simulink library "EmE_MBD_Blockset"  (R2018a)
settings: Solver=ode1  StartTime=0.0  StopTime=Inf  FixedStep=0.001  RelTol=1e-3  EnableMultiTasking=on
PostLoadFcn:
  | , if any(exist('dsrtsu_mdlpostloadfcn', 'file') == [2, 3, 6]), try dsrtsu_mdlpostloadfcn('Execute', bdroot); catch fprintf('Error in PostLoadFcn (dsrtsu_mdlpostloadfcn) for model "%s":\n %s\n', bdroot, lasterr); end, end,
undefined symbols (not defined in the file or in its folder): ENUM_TSC1_CONTROL_PURPOSE_T, gcbh, GLB_SWITCH_T
libraries: simulink x237, $bdroot x115, simulink_need_slupdate x26, MotoHawk_lib x13, simulink_extras x3
(part 7 of 11)

== system EmE_MBD_Blockset/User-Defined Functions/Snoop/CCP_ETC_SS1/Signal Data Pairing/Update Signal4 ==
  note: Configured signal information
  note: Memory address currently being configured
  PID : Inport
  Offset : Inport  Port=2
  ResetDAQ : Inport  Port=3
  Memory_Address : Inport  Port=4
  Signal_Info : Inport  Port=5
  Bus Creator : BusCreator  Inputs=6
  Bus Selector1 : BusSelector  OutputSignals=Signal_Address,Signal_Type,Signal_Conversion
  Detect Rise Positive : simulink/Logic and Bit Operations/Detect Rise Positive  vinit=0  InputProcessing=Inherited  OutDataTypeStr=uint8
  Latch w Update : Subsystem
  Latch w Update1 : Subsystem
  RS Flop-Flop Rp : Subsystem
      mask help: RS flip-flop with priority on R
  Relational Operator2 : RelationalOperator  Operator===  OutDataTypeStr=boolean  RndMeth=Nearest
  Reset Logic : Subsystem
  Terminator : Terminator
  Signal_Data_Updated : Outport
  wires:
  [PID] -> Reset Logic/1(CurrentPID)
  ResetDAQ/1 -> Reset Logic/2(ResetDAQ)
  Reset Logic/1(Reset) -> RS Flop-Flop Rp/1(Rp)
  Bus Selector1/1 -> Relational Operator2/2, Bus Creator/4  "<Signal_Address>"
  Bus Selector1/2 -> Bus Creator/5  "<Signal_Type>"
  Relational Operator2/1 -> Detect Rise Positive/1, RS Flop-Flop Rp/2(S)  "F_Signal_Defined"
  Memory_Address/1 -> Relational Operator2/1
  Signal_Info/1 -> Bus Selector1/1
  Bus Creator/1 -> Signal_Data_Updated/1
  Latch w Update/1(Latched) -> [PID], Bus Creator/1  "PID"
  Latch w Update1/1(Latched) -> Bus Creator/2  "Offset"
  Offset/1 -> Latch w Update1/2(In)
  PID/1 -> Latch w Update/2(In)
  Bus Selector1/3 -> Bus Creator/6  "<Signal_Conversion>"
  Detect Rise Positive/1 -> Latch w Update/1(f_update), Latch w Update1/1(f_update)
  RS Flop-Flop Rp/1(Q) -> Bus Creator/3  "F_Defined"
  RS Flop-Flop Rp/2(!Q) -> Terminator/1

== system EmE_MBD_Blockset/User-Defined Functions/Snoop/CCP_ETC_SS1/Signal Data Pairing/Update Signal5 ==
  note: Configured signal information
  note: Memory address currently being configured
  PID : Inport
  Offset : Inport  Port=2
  ResetDAQ : Inport  Port=3
  Memory_Address : Inport  Port=4
  Signal_Info : Inport  Port=5
  Bus Creator : BusCreator  Inputs=6
  Bus Selector1 : BusSelector  OutputSignals=Signal_Address,Signal_Type,Signal_Conversion
  Detect Rise Positive : simulink/Logic and Bit Operations/Detect Rise Positive  vinit=0  InputProcessing=Inherited  OutDataTypeStr=uint8
  Latch w Update : Subsystem
  Latch w Update1 : Subsystem
  RS Flop-Flop Rp : Subsystem
      mask help: RS flip-flop with priority on R
  Relational Operator2 : RelationalOperator  Operator===  OutDataTypeStr=boolean  RndMeth=Nearest
  Reset Logic : Subsystem
  Terminator : Terminator
  Signal_Data_Updated : Outport
  wires:
  [PID] -> Reset Logic/1(CurrentPID)
  ResetDAQ/1 -> Reset Logic/2(ResetDAQ)
  Reset Logic/1(Reset) -> RS Flop-Flop Rp/1(Rp)
  Bus Selector1/1 -> Relational Operator2/2, Bus Creator/4  "<Signal_Address>"
  Bus Selector1/2 -> Bus Creator/5  "<Signal_Type>"
  Relational Operator2/1 -> Detect Rise Positive/1, RS Flop-Flop Rp/2(S)  "F_Signal_Defined"
  Memory_Address/1 -> Relational Operator2/1
  Signal_Info/1 -> Bus Selector1/1
  Bus Creator/1 -> Signal_Data_Updated/1
  Latch w Update/1(Latched) -> [PID], Bus Creator/1  "PID"
  Latch w Update1/1(Latched) -> Bus Creator/2  "Offset"
  Offset/1 -> Latch w Update1/2(In)
  PID/1 -> Latch w Update/2(In)
  Bus Selector1/3 -> Bus Creator/6  "<Signal_Conversion>"
  Detect Rise Positive/1 -> Latch w Update/1(f_update), Latch w Update1/1(f_update)
  RS Flop-Flop Rp/1(Q) -> Bus Creator/3  "F_Defined"
  RS Flop-Flop Rp/2(!Q) -> Terminator/1

== system EmE_MBD_Blockset/User-Defined Functions/Snoop/CCP_ETC_SS1/Signal Data Pairing/Update Signal6 ==
  note: Configured signal information
  note: Memory address currently being configured
  PID : Inport
  Offset : Inport  Port=2
  ResetDAQ : Inport  Port=3
  Memory_Address : Inport  Port=4
  Signal_Info : Inport  Port=5
  Bus Creator : BusCreator  Inputs=6
  Bus Selector1 : BusSelector  OutputSignals=Signal_Address,Signal_Type,Signal_Conversion
  Detect Rise Positive : simulink/Logic and Bit Operations/Detect Rise Positive  vinit=0  InputProcessing=Inherited  OutDataTypeStr=uint8
  Latch w Update : Subsystem
  Latch w Update1 : Subsystem
  RS Flop-Flop Rp : Subsystem
      mask help: RS flip-flop with priority on R
  Relational Operator2 : RelationalOperator  Operator===  OutDataTypeStr=boolean  RndMeth=Nearest
  Reset Logic : Subsystem
  Terminator : Terminator
  Signal_Data_Updated : Outport
  wires:
  [PID] -> Reset Logic/1(CurrentPID)
  ResetDAQ/1 -> Reset Logic/2(ResetDAQ)
  Reset Logic/1(Reset) -> RS Flop-Flop Rp/1(Rp)
  Bus Selector1/1 -> Relational Operator2/2, Bus Creator/4  "<Signal_Address>"
  Bus Selector1/2 -> Bus Creator/5  "<Signal_Type>"
  Relational Operator2/1 -> Detect Rise Positive/1, RS Flop-Flop Rp/2(S)  "F_Signal_Defined"
  Memory_Address/1 -> Relational Operator2/1
  Signal_Info/1 -> Bus Selector1/1
  Bus Creator/1 -> Signal_Data_Updated/1
  Latch w Update/1(Latched) -> [PID], Bus Creator/1  "PID"
  Latch w Update1/1(Latched) -> Bus Creator/2  "Offset"
  Offset/1 -> Latch w Update1/2(In)
  PID/1 -> Latch w Update/2(In)
  Bus Selector1/3 -> Bus Creator/6  "<Signal_Conversion>"
  Detect Rise Positive/1 -> Latch w Update/1(f_update), Latch w Update1/1(f_update)
  RS Flop-Flop Rp/1(Q) -> Bus Creator/3  "F_Defined"
  RS Flop-Flop Rp/2(!Q) -> Terminator/1

== system EmE_MBD_Blockset/User-Defined Functions/Snoop/CCP_ETC_SS1/Signal Data Pairing/Update Signal7 ==
  note: Configured signal information
  note: Memory address currently being configured
  PID : Inport
  Offset : Inport  Port=2
  ResetDAQ : Inport  Port=3
  Memory_Address : Inport  Port=4
  Signal_Info : Inport  Port=5
  Bus Creator : BusCreator  Inputs=6
  Bus Selector1 : BusSelector  OutputSignals=Signal_Address,Signal_Type,Signal_Conversion
  Detect Rise Positive : simulink/Logic and Bit Operations/Detect Rise Positive  vinit=0  InputProcessing=Inherited  OutDataTypeStr=uint8
  Latch w Update : Subsystem
  Latch w Update1 : Subsystem
  RS Flop-Flop Rp : Subsystem
      mask help: RS flip-flop with priority on R
  Relational Operator2 : RelationalOperator  Operator===  OutDataTypeStr=boolean  RndMeth=Nearest
  Reset Logic : Subsystem
  Terminator : Terminator
  Signal_Data_Updated : Outport
  wires:
  [PID] -> Reset Logic/1(CurrentPID)
  ResetDAQ/1 -> Reset Logic/2(ResetDAQ)
  Reset Logic/1(Reset) -> RS Flop-Flop Rp/1(Rp)
  Bus Selector1/1 -> Relational Operator2/2, Bus Creator/4  "<Signal_Address>"
  Bus Selector1/2 -> Bus Creator/5  "<Signal_Type>"
  Relational Operator2/1 -> Detect Rise Positive/1, RS Flop-Flop Rp/2(S)  "F_Signal_Defined"
  Memory_Address/1 -> Relational Operator2/1
  Signal_Info/1 -> Bus Selector1/1
  Bus Creator/1 -> Signal_Data_Updated/1
  Latch w Update/1(Latched) -> [PID], Bus Creator/1  "PID"
  Latch w Update1/1(Latched) -> Bus Creator/2  "Offset"
  Offset/1 -> Latch w Update1/2(In)
  PID/1 -> Latch w Update/2(In)
  Bus Selector1/3 -> Bus Creator/6  "<Signal_Conversion>"
  Detect Rise Positive/1 -> Latch w Update/1(f_update), Latch w Update1/1(f_update)
  RS Flop-Flop Rp/1(Q) -> Bus Creator/3  "F_Defined"
  RS Flop-Flop Rp/2(!Q) -> Terminator/1

== system EmE_MBD_Blockset/User-Defined Functions/Snoop/CCP_ETC_SS1/Signal Data Pairing/Update Signal8 ==
  note: Configured signal information
  note: Memory address currently being configured
  PID : Inport
  Offset : Inport  Port=2
  ResetDAQ : Inport  Port=3
  Memory_Address : Inport  Port=4
  Signal_Info : Inport  Port=5
  Bus Creator : BusCreator  Inputs=6
  Bus Selector1 : BusSelector  OutputSignals=Signal_Address,Signal_Type,Signal_Conversion
  Detect Rise Positive : simulink/Logic and Bit Operations/Detect Rise Positive  vinit=0  InputProcessing=Inherited  OutDataTypeStr=uint8
  Latch w Update : Subsystem
  Latch w Update1 : Subsystem
  RS Flop-Flop Rp : Subsystem
      mask help: RS flip-flop with priority on R
  Relational Operator2 : RelationalOperator  Operator===  OutDataTypeStr=boolean  RndMeth=Nearest
  Reset Logic : Subsystem
  Terminator : Terminator
  Signal_Data_Updated : Outport
  wires:
  [PID] -> Reset Logic/1(CurrentPID)
  ResetDAQ/1 -> Reset Logic/2(ResetDAQ)
  Reset Logic/1(Reset) -> RS Flop-Flop Rp/1(Rp)
  Bus Selector1/1 -> Relational Operator2/2, Bus Creator/4  "<Signal_Address>"
  Bus Selector1/2 -> Bus Creator/5  "<Signal_Type>"
  Relational Operator2/1 -> Detect Rise Positive/1, RS Flop-Flop Rp/2(S)  "F_Signal_Defined"
  Memory_Address/1 -> Relational Operator2/1
  Signal_Info/1 -> Bus Selector1/1
  Bus Creator/1 -> Signal_Data_Updated/1
  Latch w Update/1(Latched) -> [PID], Bus Creator/1  "PID"
  Latch w Update1/1(Latched) -> Bus Creator/2  "Offset"
  Offset/1 -> Latch w Update1/2(In)
  PID/1 -> Latch w Update/2(In)
  Bus Selector1/3 -> Bus Creator/6  "<Signal_Conversion>"
  Detect Rise Positive/1 -> Latch w Update/1(f_update), Latch w Update1/1(f_update)
  RS Flop-Flop Rp/1(Q) -> Bus Creator/3  "F_Defined"
  RS Flop-Flop Rp/2(!Q) -> Terminator/1

== system EmE_MBD_Blockset/User-Defined Functions/Snoop/CCP_ETC_SS1/Signal Data Pairing/Update Signal9 ==
  note: Configured signal information
  note: Memory address currently being configured
  PID : Inport
  Offset : Inport  Port=2
  ResetDAQ : Inport  Port=3
  Memory_Address : Inport  Port=4
  Signal_Info : Inport  Port=5
  Bus Creator : BusCreator  Inputs=6
  Bus Selector1 : BusSelector  OutputSignals=Signal_Address,Signal_Type,Signal_Conversion
  Detect Rise Positive : simulink/Logic and Bit Operations/Detect Rise Positive  vinit=0  InputProcessing=Inherited  OutDataTypeStr=uint8
  Latch w Update : Subsystem
  Latch w Update1 : Subsystem
  RS Flop-Flop Rp : Subsystem
      mask help: RS flip-flop with priority on R
  Relational Operator2 : RelationalOperator  Operator===  OutDataTypeStr=boolean  RndMeth=Nearest
  Reset Logic : Subsystem
  Terminator : Terminator
  Signal_Data_Updated : Outport
  wires:
  [PID] -> Reset Logic/1(CurrentPID)
  ResetDAQ/1 -> Reset Logic/2(ResetDAQ)
  Reset Logic/1(Reset) -> RS Flop-Flop Rp/1(Rp)
  Bus Selector1/1 -> Relational Operator2/2, Bus Creator/4  "<Signal_Address>"
  Bus Selector1/2 -> Bus Creator/5  "<Signal_Type>"
  Relational Operator2/1 -> Detect Rise Positive/1, RS Flop-Flop Rp/2(S)  "F_Signal_Defined"
  Memory_Address/1 -> Relational Operator2/1
  Signal_Info/1 -> Bus Selector1/1
  Bus Creator/1 -> Signal_Data_Updated/1
  Latch w Update/1(Latched) -> [PID], Bus Creator/1  "PID"
  Latch w Update1/1(Latched) -> Bus Creator/2  "Offset"
  Offset/1 -> Latch w Update1/2(In)
  PID/1 -> Latch w Update/2(In)
  Bus Selector1/3 -> Bus Creator/6  "<Signal_Conversion>"
  Detect Rise Positive/1 -> Latch w Update/1(f_update), Latch w Update1/1(f_update)
  RS Flop-Flop Rp/1(Q) -> Bus Creator/3  "F_Defined"
  RS Flop-Flop Rp/2(!Q) -> Terminator/1

== system EmE_MBD_Blockset/User-Defined Functions/Snoop/CCP_ETC_SS2/CCP_Parameter_Decode/Decode_Signal1 ==
  PID : Inport
  Data : Inport  Port=2
  Signal_Info : Inport  Port=3
  Bus Selector : BusSelector  OutputSignals=Offset,Signal_Address,Signal_Type,Signal_Conversion,PID,F_Defined
  Isolate Data : Subsystem
  Relational Operator : RelationalOperator  Operator===  OutDataTypeStr=boolean  RndMeth=Nearest
  Signal Decode : Subsystem
  Switch2 : Switch  Criteria=u2 ~= 0
  Terminator : Terminator
  Terminator1 : Terminator
  Unit Delay : UnitDelay  SampleTime=-1
  Signal : Outport
  wires:
  Bus Selector/2 -> Terminator/1  "<Signal_Address>"
  Switch2/1 -> Signal/1, Unit Delay/1
  Bus Selector/6 -> Terminator1/1  "<F_Defined>"
  Signal Decode/1(Out1) -> Switch2/1
  Unit Delay/1 -> Switch2/3
  Bus Selector/1 -> Isolate Data/1(Offset)  "<Offset>"
  PID/1 -> Relational Operator/2
  Relational Operator/1 -> Switch2/2
  Data/1 -> Isolate Data/2(Data)
  Bus Selector/5 -> Relational Operator/1  "<PID>"
  Bus Selector/3 -> Signal Decode/2(Type), Isolate Data/3(Type)  "<Signal_Type>"
  Bus Selector/4 -> Signal Decode/3(Coversion)  "<Signal_Conversion>"
  Signal_Info/1 -> Bus Selector/1
  Isolate Data/1(Raw32) -> Signal Decode/1(Raw32)

== system EmE_MBD_Blockset/User-Defined Functions/Snoop/CCP_ETC_SS2/CCP_Parameter_Decode/Decode_Signal10 ==
  PID : Inport
  Data : Inport  Port=2
  Signal_Info : Inport  Port=3
  Bus Selector : BusSelector  OutputSignals=Offset,Signal_Address,Signal_Type,Signal_Conversion,PID,F_Defined
  Isolate Data : Subsystem
  Relational Operator : RelationalOperator  Operator===  OutDataTypeStr=boolean  RndMeth=Nearest
  Signal Decode : Subsystem
  Switch2 : Switch  Criteria=u2 ~= 0
  Terminator : Terminator
  Terminator1 : Terminator
  Unit Delay : UnitDelay  SampleTime=-1
  Signal : Outport
  wires:
  Isolate Data/1(Raw32) -> Signal Decode/1(Raw32)
  Signal_Info/1 -> Bus Selector/1
  Bus Selector/4 -> Signal Decode/3(Coversion)  "<Signal_Conversion>"
  Bus Selector/3 -> Isolate Data/3(Type), Signal Decode/2(Type)  "<Signal_Type>"
  Bus Selector/5 -> Relational Operator/1  "<PID>"
  Data/1 -> Isolate Data/2(Data)
  Relational Operator/1 -> Switch2/2
  PID/1 -> Relational Operator/2
  Bus Selector/1 -> Isolate Data/1(Offset)  "<Offset>"
  Unit Delay/1 -> Switch2/3
  Signal Decode/1(Out1) -> Switch2/1
  Bus Selector/6 -> Terminator1/1  "<F_Defined>"
  Switch2/1 -> Unit Delay/1, Signal/1
  Bus Selector/2 -> Terminator/1  "<Signal_Address>"

== system EmE_MBD_Blockset/User-Defined Functions/Snoop/CCP_ETC_SS2/CCP_Parameter_Decode/Decode_Signal11 ==
  PID : Inport
  Data : Inport  Port=2
  Signal_Info : Inport  Port=3
  Bus Selector : BusSelector  OutputSignals=Offset,Signal_Address,Signal_Type,Signal_Conversion,PID,F_Defined
  Isolate Data : Subsystem
  Relational Operator : RelationalOperator  Operator===  OutDataTypeStr=boolean  RndMeth=Nearest
  Signal Decode : Subsystem
  Switch2 : Switch  Criteria=u2 ~= 0
  Terminator : Terminator
  Terminator1 : Terminator
  Unit Delay : UnitDelay  SampleTime=-1
  Signal : Outport
  wires:
  Bus Selector/2 -> Terminator/1  "<Signal_Address>"
  Switch2/1 -> Signal/1, Unit Delay/1
  Bus Selector/6 -> Terminator1/1  "<F_Defined>"
  Signal Decode/1(Out1) -> Switch2/1
  Unit Delay/1 -> Switch2/3
  Bus Selector/1 -> Isolate Data/1(Offset)  "<Offset>"
  PID/1 -> Relational Operator/2
  Relational Operator/1 -> Switch2/2
  Data/1 -> Isolate Data/2(Data)
  Bus Selector/5 -> Relational Operator/1  "<PID>"
  Bus Selector/3 -> Signal Decode/2(Type), Isolate Data/3(Type)  "<Signal_Type>"
  Bus Selector/4 -> Signal Decode/3(Coversion)  "<Signal_Conversion>"
  Signal_Info/1 -> Bus Selector/1
  Isolate Data/1(Raw32) -> Signal Decode/1(Raw32)

== system EmE_MBD_Blockset/User-Defined Functions/Snoop/CCP_ETC_SS2/CCP_Parameter_Decode/Decode_Signal12 ==
  PID : Inport
  Data : Inport  Port=2
  Signal_Info : Inport  Port=3
  Bus Selector : BusSelector  OutputSignals=Offset,Signal_Address,Signal_Type,Signal_Conversion,PID,F_Defined
  Isolate Data : Subsystem
  Relational Operator : RelationalOperator  Operator===  OutDataTypeStr=boolean  RndMeth=Nearest
  Signal Decode : Subsystem
  Switch2 : Switch  Criteria=u2 ~= 0
  Terminator : Terminator
  Terminator1 : Terminator
  Unit Delay : UnitDelay  SampleTime=-1
  Signal : Outport
  wires:
  Isolate Data/1(Raw32) -> Signal Decode/1(Raw32)
  Signal_Info/1 -> Bus Selector/1
  Bus Selector/4 -> Signal Decode/3(Coversion)  "<Signal_Conversion>"
  Bus Selector/3 -> Isolate Data/3(Type), Signal Decode/2(Type)  "<Signal_Type>"
  Bus Selector/5 -> Relational Operator/1  "<PID>"
  Data/1 -> Isolate Data/2(Data)
  Relational Operator/1 -> Switch2/2
  PID/1 -> Relational Operator/2
  Bus Selector/1 -> Isolate Data/1(Offset)  "<Offset>"
  Unit Delay/1 -> Switch2/3
  Signal Decode/1(Out1) -> Switch2/1
  Bus Selector/6 -> Terminator1/1  "<F_Defined>"
  Switch2/1 -> Unit Delay/1, Signal/1
  Bus Selector/2 -> Terminator/1  "<Signal_Address>"

== system EmE_MBD_Blockset/User-Defined Functions/Snoop/CCP_ETC_SS2/CCP_Parameter_Decode/Decode_Signal2 ==
  PID : Inport
  Data : Inport  Port=2
  Signal_Info : Inport  Port=3
  Bus Selector : BusSelector  OutputSignals=Offset,Signal_Address,Signal_Type,Signal_Conversion,PID,F_Defined
  Isolate Data : Subsystem
  Relational Operator : RelationalOperator  Operator===  OutDataTypeStr=boolean  RndMeth=Nearest
  Signal Decode : Subsystem
  Switch2 : Switch  Criteria=u2 ~= 0
  Terminator : Terminator
  Terminator1 : Terminator
  Unit Delay : UnitDelay  SampleTime=-1
  Signal : Outport
  wires:
  Isolate Data/1(Raw32) -> Signal Decode/1(Raw32)
  Signal_Info/1 -> Bus Selector/1
  Bus Selector/4 -> Signal Decode/3(Coversion)  "<Signal_Conversion>"
  Bus Selector/3 -> Isolate Data/3(Type), Signal Decode/2(Type)  "<Signal_Type>"
  Bus Selector/5 -> Relational Operator/1  "<PID>"
  Data/1 -> Isolate Data/2(Data)
  Relational Operator/1 -> Switch2/2
  PID/1 -> Relational Operator/2
  Bus Selector/1 -> Isolate Data/1(Offset)  "<Offset>"
  Unit Delay/1 -> Switch2/3
  Signal Decode/1(Out1) -> Switch2/1
  Bus Selector/6 -> Terminator1/1  "<F_Defined>"
  Switch2/1 -> Unit Delay/1, Signal/1
  Bus Selector/2 -> Terminator/1  "<Signal_Address>"

== system EmE_MBD_Blockset/User-Defined Functions/Snoop/CCP_ETC_SS2/CCP_Parameter_Decode/Decode_Signal3 ==
  PID : Inport
  Data : Inport  Port=2
  Signal_Info : Inport  Port=3
  Bus Selector : BusSelector  OutputSignals=Offset,Signal_Address,Signal_Type,Signal_Conversion,PID,F_Defined
  Isolate Data : Subsystem
  Relational Operator : RelationalOperator  Operator===  OutDataTypeStr=boolean  RndMeth=Nearest
  Signal Decode : Subsystem
  Switch2 : Switch  Criteria=u2 ~= 0
  Terminator : Terminator
  Terminator1 : Terminator
  Unit Delay : UnitDelay  SampleTime=-1
  Signal : Outport
  wires:
  Bus Selector/2 -> Terminator/1  "<Signal_Address>"
  Switch2/1 -> Signal/1, Unit Delay/1
  Bus Selector/6 -> Terminator1/1  "<F_Defined>"
  Signal Decode/1(Out1) -> Switch2/1
  Unit Delay/1 -> Switch2/3
  Bus Selector/1 -> Isolate Data/1(Offset)  "<Offset>"
  PID/1 -> Relational Operator/2
  Relational Operator/1 -> Switch2/2
  Data/1 -> Isolate Data/2(Data)
  Bus Selector/5 -> Relational Operator/1  "<PID>"
  Bus Selector/3 -> Signal Decode/2(Type), Isolate Data/3(Type)  "<Signal_Type>"
  Bus Selector/4 -> Signal Decode/3(Coversion)  "<Signal_Conversion>"
  Signal_Info/1 -> Bus Selector/1
  Isolate Data/1(Raw32) -> Signal Decode/1(Raw32)

== system EmE_MBD_Blockset/User-Defined Functions/Snoop/CCP_ETC_SS2/CCP_Parameter_Decode/Decode_Signal4 ==
  PID : Inport
  Data : Inport  Port=2
  Signal_Info : Inport  Port=3
  Bus Selector : BusSelector  OutputSignals=Offset,Signal_Address,Signal_Type,Signal_Conversion,PID,F_Defined
  Isolate Data : Subsystem
  Relational Operator : RelationalOperator  Operator===  OutDataTypeStr=boolean  RndMeth=Nearest
  Signal Decode : Subsystem
  Switch2 : Switch  Criteria=u2 ~= 0
  Terminator : Terminator
  Terminator1 : Terminator
  Unit Delay : UnitDelay  SampleTime=-1
  Signal : Outport
  wires:
  Isolate Data/1(Raw32) -> Signal Decode/1(Raw32)
  Signal_Info/1 -> Bus Selector/1
  Bus Selector/4 -> Signal Decode/3(Coversion)  "<Signal_Conversion>"
  Bus Selector/3 -> Isolate Data/3(Type), Signal Decode/2(Type)  "<Signal_Type>"
  Bus Selector/5 -> Relational Operator/1  "<PID>"
  Data/1 -> Isolate Data/2(Data)
  Relational Operator/1 -> Switch2/2
  PID/1 -> Relational Operator/2
  Bus Selector/1 -> Isolate Data/1(Offset)  "<Offset>"
  Unit Delay/1 -> Switch2/3
  Signal Decode/1(Out1) -> Switch2/1
  Bus Selector/6 -> Terminator1/1  "<F_Defined>"
  Switch2/1 -> Unit Delay/1, Signal/1
  Bus Selector/2 -> Terminator/1  "<Signal_Address>"

== system EmE_MBD_Blockset/User-Defined Functions/Snoop/CCP_ETC_SS2/CCP_Parameter_Decode/Decode_Signal5 ==
  PID : Inport
  Data : Inport  Port=2
  Signal_Info : Inport  Port=3
  Bus Selector : BusSelector  OutputSignals=Offset,Signal_Address,Signal_Type,Signal_Conversion,PID,F_Defined
  Isolate Data : Subsystem
  Relational Operator : RelationalOperator  Operator===  OutDataTypeStr=boolean  RndMeth=Nearest
  Signal Decode : Subsystem
  Switch2 : Switch  Criteria=u2 ~= 0
  Terminator : Terminator
  Terminator1 : Terminator
  Unit Delay : UnitDelay  SampleTime=-1
  Signal : Outport
  wires:
  Bus Selector/2 -> Terminator/1  "<Signal_Address>"
  Switch2/1 -> Signal/1, Unit Delay/1
  Bus Selector/6 -> Terminator1/1  "<F_Defined>"
  Signal Decode/1(Out1) -> Switch2/1
  Unit Delay/1 -> Switch2/3
  Bus Selector/1 -> Isolate Data/1(Offset)  "<Offset>"
  PID/1 -> Relational Operator/2
  Relational Operator/1 -> Switch2/2
  Data/1 -> Isolate Data/2(Data)
  Bus Selector/5 -> Relational Operator/1  "<PID>"
  Bus Selector/3 -> Signal Decode/2(Type), Isolate Data/3(Type)  "<Signal_Type>"
  Bus Selector/4 -> Signal Decode/3(Coversion)  "<Signal_Conversion>"
  Signal_Info/1 -> Bus Selector/1
  Isolate Data/1(Raw32) -> Signal Decode/1(Raw32)

== system EmE_MBD_Blockset/User-Defined Functions/Snoop/CCP_ETC_SS2/CCP_Parameter_Decode/Decode_Signal6 ==
  PID : Inport
  Data : Inport  Port=2
  Signal_Info : Inport  Port=3
  Bus Selector : BusSelector  OutputSignals=Offset,Signal_Address,Signal_Type,Signal_Conversion,PID,F_Defined
  Isolate Data : Subsystem
  Relational Operator : RelationalOperator  Operator===  OutDataTypeStr=boolean  RndMeth=Nearest
  Signal Decode : Subsystem
  Switch2 : Switch  Criteria=u2 ~= 0
  Terminator : Terminator
  Terminator1 : Terminator
  Unit Delay : UnitDelay  SampleTime=-1
  Signal : Outport
  wires:
  Isolate Data/1(Raw32) -> Signal Decode/1(Raw32)
  Signal_Info/1 -> Bus Selector/1
  Bus Selector/4 -> Signal Decode/3(Coversion)  "<Signal_Conversion>"
  Bus Selector/3 -> Isolate Data/3(Type), Signal Decode/2(Type)  "<Signal_Type>"
  Bus Selector/5 -> Relational Operator/1  "<PID>"
  Data/1 -> Isolate Data/2(Data)
  Relational Operator/1 -> Switch2/2
  PID/1 -> Relational Operator/2
  Bus Selector/1 -> Isolate Data/1(Offset)  "<Offset>"
  Unit Delay/1 -> Switch2/3
  Signal Decode/1(Out1) -> Switch2/1
  Bus Selector/6 -> Terminator1/1  "<F_Defined>"
  Switch2/1 -> Unit Delay/1, Signal/1
  Bus Selector/2 -> Terminator/1  "<Signal_Address>"

== system EmE_MBD_Blockset/User-Defined Functions/Snoop/CCP_ETC_SS2/CCP_Parameter_Decode/Decode_Signal7 ==
  PID : Inport
  Data : Inport  Port=2
  Signal_Info : Inport  Port=3
  Bus Selector : BusSelector  OutputSignals=Offset,Signal_Address,Signal_Type,Signal_Conversion,PID,F_Defined
  Isolate Data : Subsystem
  Relational Operator : RelationalOperator  Operator===  OutDataTypeStr=boolean  RndMeth=Nearest
  Signal Decode : Subsystem
  Switch2 : Switch  Criteria=u2 ~= 0
  Terminator : Terminator
  Terminator1 : Terminator
  Unit Delay : UnitDelay  SampleTime=-1
  Signal : Outport
  wires:
  Bus Selector/2 -> Terminator/1  "<Signal_Address>"
  Switch2/1 -> Signal/1, Unit Delay/1
  Bus Selector/6 -> Terminator1/1  "<F_Defined>"
  Signal Decode/1(Out1) -> Switch2/1
  Unit Delay/1 -> Switch2/3
  Bus Selector/1 -> Isolate Data/1(Offset)  "<Offset>"
  PID/1 -> Relational Operator/2
  Relational Operator/1 -> Switch2/2
  Data/1 -> Isolate Data/2(Data)
  Bus Selector/5 -> Relational Operator/1  "<PID>"
  Bus Selector/3 -> Signal Decode/2(Type), Isolate Data/3(Type)  "<Signal_Type>"
  Bus Selector/4 -> Signal Decode/3(Coversion)  "<Signal_Conversion>"
  Signal_Info/1 -> Bus Selector/1
  Isolate Data/1(Raw32) -> Signal Decode/1(Raw32)

== system EmE_MBD_Blockset/User-Defined Functions/Snoop/CCP_ETC_SS2/CCP_Parameter_Decode/Decode_Signal8 ==
  PID : Inport
  Data : Inport  Port=2
  Signal_Info : Inport  Port=3
  Bus Selector : BusSelector  OutputSignals=Offset,Signal_Address,Signal_Type,Signal_Conversion,PID,F_Defined
  Isolate Data : Subsystem
  Relational Operator : RelationalOperator  Operator===  OutDataTypeStr=boolean  RndMeth=Nearest
  Signal Decode : Subsystem
  Switch2 : Switch  Criteria=u2 ~= 0
  Terminator : Terminator
  Terminator1 : Terminator
  Unit Delay : UnitDelay  SampleTime=-1
  Signal : Outport
  wires:
  Isolate Data/1(Raw32) -> Signal Decode/1(Raw32)
  Signal_Info/1 -> Bus Selector/1
  Bus Selector/4 -> Signal Decode/3(Coversion)  "<Signal_Conversion>"
  Bus Selector/3 -> Isolate Data/3(Type), Signal Decode/2(Type)  "<Signal_Type>"
  Bus Selector/5 -> Relational Operator/1  "<PID>"
  Data/1 -> Isolate Data/2(Data)
  Relational Operator/1 -> Switch2/2
  PID/1 -> Relational Operator/2
  Bus Selector/1 -> Isolate Data/1(Offset)  "<Offset>"
  Unit Delay/1 -> Switch2/3
  Signal Decode/1(Out1) -> Switch2/1
  Bus Selector/6 -> Terminator1/1  "<F_Defined>"
  Switch2/1 -> Unit Delay/1, Signal/1
  Bus Selector/2 -> Terminator/1  "<Signal_Address>"

== system EmE_MBD_Blockset/User-Defined Functions/Snoop/CCP_ETC_SS2/CCP_Parameter_Decode/Decode_Signal9 ==
  PID : Inport
  Data : Inport  Port=2
  Signal_Info : Inport  Port=3
  Bus Selector : BusSelector  OutputSignals=Offset,Signal_Address,Signal_Type,Signal_Conversion,PID,F_Defined
  Isolate Data : Subsystem
  Relational Operator : RelationalOperator  Operator===  OutDataTypeStr=boolean  RndMeth=Nearest
  Signal Decode : Subsystem
  Switch2 : Switch  Criteria=u2 ~= 0
  Terminator : Terminator
  Terminator1 : Terminator
  Unit Delay : UnitDelay  SampleTime=-1
  Signal : Outport
  wires:
  Bus Selector/2 -> Terminator/1  "<Signal_Address>"
  Switch2/1 -> Signal/1, Unit Delay/1
  Bus Selector/6 -> Terminator1/1  "<F_Defined>"
  Signal Decode/1(Out1) -> Switch2/1
  Unit Delay/1 -> Switch2/3
  Bus Selector/1 -> Isolate Data/1(Offset)  "<Offset>"
  PID/1 -> Relational Operator/2
  Relational Operator/1 -> Switch2/2
  Data/1 -> Isolate Data/2(Data)
  Bus Selector/5 -> Relational Operator/1  "<PID>"
  Bus Selector/3 -> Signal Decode/2(Type), Isolate Data/3(Type)  "<Signal_Type>"
  Bus Selector/4 -> Signal Decode/3(Coversion)  "<Signal_Conversion>"
  Signal_Info/1 -> Bus Selector/1
  Isolate Data/1(Raw32) -> Signal Decode/1(Raw32)

== system EmE_MBD_Blockset/User-Defined Functions/Snoop/CCP_ETC_SS1/Signal Data Pairing/Update Signal1/Latch w Update ==
  f_update : Inport
  In : Inport  Port=2
  Switch : Switch  Criteria=u2 ~= 0
  Unit Delay1 : UnitDelay  SampleTime=-1
  Latched : Outport
  wires:
  f_update/1 -> Switch/2
  In/1 -> Switch/1
  Switch/1 -> Latched/1, Unit Delay1/1
  Unit Delay1/1 -> Switch/3

== system EmE_MBD_Blockset/User-Defined Functions/Snoop/CCP_ETC_SS1/Signal Data Pairing/Update Signal1/Latch w Update1 ==
  f_update : Inport
  In : Inport  Port=2
  Switch : Switch  Criteria=u2 ~= 0
  Unit Delay1 : UnitDelay  SampleTime=-1
  Latched : Outport
  wires:
  Unit Delay1/1 -> Switch/3
  Switch/1 -> Unit Delay1/1, Latched/1
  In/1 -> Switch/1
  f_update/1 -> Switch/2

== system EmE_MBD_Blockset/User-Defined Functions/Snoop/CCP_ETC_SS1/Signal Data Pairing/Update Signal1/RS Flop-Flop Rp ==
  Rp : Inport
  S : Inport  Port=2
  Logical Operator : Logic  Operator=NOT  AllPortsSameDT=off
  Logical Operator1 : Logic  AllPortsSameDT=off
  Logical Operator2 : Logic  Operator=OR  AllPortsSameDT=off
  Logical Operator3 : Logic  Operator=NOT  AllPortsSameDT=off
  Unit Delay : UnitDelay  SampleTime=-1
  Q : Outport
  !Q : Outport  Port=2
  wires:
  Logical Operator/1 -> Logical Operator1/1
  Logical Operator2/1 -> Logical Operator1/2
  Logical Operator1/1 -> Q/1, Logical Operator3/1, Unit Delay/1
  Unit Delay/1 -> Logical Operator2/2
  Logical Operator3/1 -> !Q/1
  Rp/1 -> Logical Operator/1
  S/1 -> Logical Operator2/1

== system EmE_MBD_Blockset/User-Defined Functions/Snoop/CCP_ETC_SS1/Signal Data Pairing/Update Signal1/Reset Logic ==
  CurrentPID : Inport
  ResetDAQ : Inport  Port=2
  CCP_SNOOP_DAQSIZE : Constant  Value=16  OutDataTypeStr=uint8
  CCP_SNOOP_FIRSTPID : Constant  Value=64  OutDataTypeStr=uint8
  Divide : Product  Inputs=*/
  Logical Operator : Logic  Operator=OR  AllPortsSameDT=off  OutDataTypeStr=boolean
  Relational Operator : RelationalOperator  Operator===  OutDataTypeStr=boolean  RndMeth=Nearest
  Relational Operator1 : RelationalOperator  Operator===  OutDataTypeStr=boolean  RndMeth=Nearest
  Reset ALL : Constant  Value=250  OutDataTypeStr=uint8
  Subtract : Sum  Inputs=+-
  Reset : Outport
  wires:
  CurrentPID/1 -> Subtract/1
  Subtract/1 -> Divide/1
  CCP_SNOOP_DAQSIZE/1 -> Divide/2
  Divide/1 -> Relational Operator/1  "CurrentDAQ"
  ResetDAQ/1 -> Relational Operator/2, Relational Operator1/1
  Reset ALL/1 -> Relational Operator1/2
  Relational Operator/1 -> Logical Operator/1
  Relational Operator1/1 -> Logical Operator/2
  Logical Operator/1 -> Reset/1
  CCP_SNOOP_FIRSTPID/1 -> Subtract/2

== system EmE_MBD_Blockset/User-Defined Functions/Snoop/CCP_ETC_SS1/Signal Data Pairing/Update Signal10/Latch w Update ==
  f_update : Inport
  In : Inport  Port=2
  Switch : Switch  Criteria=u2 ~= 0
  Unit Delay1 : UnitDelay  SampleTime=-1
  Latched : Outport
  wires:
  Unit Delay1/1 -> Switch/3
  Switch/1 -> Unit Delay1/1, Latched/1
  In/1 -> Switch/1
  f_update/1 -> Switch/2

== system EmE_MBD_Blockset/User-Defined Functions/Snoop/CCP_ETC_SS1/Signal Data Pairing/Update Signal10/Latch w Update1 ==
  f_update : Inport
  In : Inport  Port=2
  Switch : Switch  Criteria=u2 ~= 0
  Unit Delay1 : UnitDelay  SampleTime=-1
  Latched : Outport
  wires:
  f_update/1 -> Switch/2
  In/1 -> Switch/1
  Switch/1 -> Latched/1, Unit Delay1/1
  Unit Delay1/1 -> Switch/3

== system EmE_MBD_Blockset/User-Defined Functions/Snoop/CCP_ETC_SS1/Signal Data Pairing/Update Signal10/RS Flop-Flop Rp ==
  Rp : Inport
  S : Inport  Port=2
  Logical Operator : Logic  Operator=NOT  AllPortsSameDT=off
  Logical Operator1 : Logic  AllPortsSameDT=off
  Logical Operator2 : Logic  Operator=OR  AllPortsSameDT=off
  Logical Operator3 : Logic  Operator=NOT  AllPortsSameDT=off
  Unit Delay : UnitDelay  SampleTime=-1
  Q : Outport
  !Q : Outport  Port=2
  wires:
  S/1 -> Logical Operator2/1
  Rp/1 -> Logical Operator/1
  Logical Operator3/1 -> !Q/1
  Unit Delay/1 -> Logical Operator2/2
  Logical Operator1/1 -> Unit Delay/1, Logical Operator3/1, Q/1
  Logical Operator2/1 -> Logical Operator1/2
  Logical Operator/1 -> Logical Operator1/1

== system EmE_MBD_Blockset/User-Defined Functions/Snoop/CCP_ETC_SS1/Signal Data Pairing/Update Signal10/Reset Logic ==
  CurrentPID : Inport
  ResetDAQ : Inport  Port=2
  CCP_SNOOP_DAQSIZE : Constant  Value=16  OutDataTypeStr=uint8
  CCP_SNOOP_FIRSTPID : Constant  Value=64  OutDataTypeStr=uint8
  Divide : Product  Inputs=*/
  Logical Operator : Logic  Operator=OR  AllPortsSameDT=off  OutDataTypeStr=boolean
  Relational Operator : RelationalOperator  Operator===  OutDataTypeStr=boolean  RndMeth=Nearest
  Relational Operator1 : RelationalOperator  Operator===  OutDataTypeStr=boolean  RndMeth=Nearest
  Reset ALL : Constant  Value=250  OutDataTypeStr=uint8
  Subtract : Sum  Inputs=+-
  Reset : Outport
  wires:
  CCP_SNOOP_FIRSTPID/1 -> Subtract/2
  Logical Operator/1 -> Reset/1
  Relational Operator1/1 -> Logical Operator/2
  Relational Operator/1 -> Logical Operator/1
  Reset ALL/1 -> Relational Operator1/2
  ResetDAQ/1 -> Relational Operator1/1, Relational Operator/2
  Divide/1 -> Relational Operator/1  "CurrentDAQ"
  CCP_SNOOP_DAQSIZE/1 -> Divide/2
  Subtract/1 -> Divide/1
  CurrentPID/1 -> Subtract/1

== system EmE_MBD_Blockset/User-Defined Functions/Snoop/CCP_ETC_SS1/Signal Data Pairing/Update Signal11/Latch w Update ==
  f_update : Inport
  In : Inport  Port=2
  Switch : Switch  Criteria=u2 ~= 0
  Unit Delay1 : UnitDelay  SampleTime=-1
  Latched : Outport
  wires:
  Unit Delay1/1 -> Switch/3
  Switch/1 -> Unit Delay1/1, Latched/1
  In/1 -> Switch/1
  f_update/1 -> Switch/2

== system EmE_MBD_Blockset/User-Defined Functions/Snoop/CCP_ETC_SS1/Signal Data Pairing/Update Signal11/Latch w Update1 ==
  f_update : Inport
  In : Inport  Port=2
  Switch : Switch  Criteria=u2 ~= 0
  Unit Delay1 : UnitDelay  SampleTime=-1
  Latched : Outport
  wires:
  f_update/1 -> Switch/2
  In/1 -> Switch/1
  Switch/1 -> Latched/1, Unit Delay1/1
  Unit Delay1/1 -> Switch/3

== system EmE_MBD_Blockset/User-Defined Functions/Snoop/CCP_ETC_SS1/Signal Data Pairing/Update Signal11/RS Flop-Flop Rp ==
  Rp : Inport
  S : Inport  Port=2
  Logical Operator : Logic  Operator=NOT  AllPortsSameDT=off
  Logical Operator1 : Logic  AllPortsSameDT=off
  Logical Operator2 : Logic  Operator=OR  AllPortsSameDT=off
  Logical Operator3 : Logic  Operator=NOT  AllPortsSameDT=off
  Unit Delay : UnitDelay  SampleTime=-1
  Q : Outport
  !Q : Outport  Port=2
  wires:
  S/1 -> Logical Operator2/1
  Rp/1 -> Logical Operator/1
  Logical Operator3/1 -> !Q/1
  Unit Delay/1 -> Logical Operator2/2
  Logical Operator1/1 -> Unit Delay/1, Logical Operator3/1, Q/1
  Logical Operator2/1 -> Logical Operator1/2
  Logical Operator/1 -> Logical Operator1/1

== system EmE_MBD_Blockset/User-Defined Functions/Snoop/CCP_ETC_SS1/Signal Data Pairing/Update Signal11/Reset Logic ==
  CurrentPID : Inport
  ResetDAQ : Inport  Port=2
  CCP_SNOOP_DAQSIZE : Constant  Value=16  OutDataTypeStr=uint8
  CCP_SNOOP_FIRSTPID : Constant  Value=64  OutDataTypeStr=uint8
  Divide : Product  Inputs=*/
  Logical Operator : Logic  Operator=OR  AllPortsSameDT=off  OutDataTypeStr=boolean
  Relational Operator : RelationalOperator  Operator===  OutDataTypeStr=boolean  RndMeth=Nearest
  Relational Operator1 : RelationalOperator  Operator===  OutDataTypeStr=boolean  RndMeth=Nearest
  Reset ALL : Constant  Value=250  OutDataTypeStr=uint8
  Subtract : Sum  Inputs=+-
  Reset : Outport
  wires:
  CCP_SNOOP_FIRSTPID/1 -> Subtract/2
  Logical Operator/1 -> Reset/1
  Relational Operator1/1 -> Logical Operator/2
  Relational Operator/1 -> Logical Operator/1
  Reset ALL/1 -> Relational Operator1/2
  ResetDAQ/1 -> Relational Operator1/1, Relational Operator/2
  Divide/1 -> Relational Operator/1  "CurrentDAQ"
  CCP_SNOOP_DAQSIZE/1 -> Divide/2
  Subtract/1 -> Divide/1
  CurrentPID/1 -> Subtract/1

== system EmE_MBD_Blockset/User-Defined Functions/Snoop/CCP_ETC_SS1/Signal Data Pairing/Update Signal12/Latch w Update ==
  f_update : Inport
  In : Inport  Port=2
  Switch : Switch  Criteria=u2 ~= 0
  Unit Delay1 : UnitDelay  SampleTime=-1
  Latched : Outport
  wires:
  Unit Delay1/1 -> Switch/3
  Switch/1 -> Unit Delay1/1, Latched/1
  In/1 -> Switch/1
  f_update/1 -> Switch/2

== system EmE_MBD_Blockset/User-Defined Functions/Snoop/CCP_ETC_SS1/Signal Data Pairing/Update Signal12/Latch w Update1 ==
  f_update : Inport
  In : Inport  Port=2
  Switch : Switch  Criteria=u2 ~= 0
  Unit Delay1 : UnitDelay  SampleTime=-1
  Latched : Outport
  wires:
  f_update/1 -> Switch/2
  In/1 -> Switch/1
  Switch/1 -> Latched/1, Unit Delay1/1
  Unit Delay1/1 -> Switch/3

== system EmE_MBD_Blockset/User-Defined Functions/Snoop/CCP_ETC_SS1/Signal Data Pairing/Update Signal12/RS Flop-Flop Rp ==
  Rp : Inport
  S : Inport  Port=2
  Logical Operator : Logic  Operator=NOT  AllPortsSameDT=off
  Logical Operator1 : Logic  AllPortsSameDT=off
  Logical Operator2 : Logic  Operator=OR  AllPortsSameDT=off
  Logical Operator3 : Logic  Operator=NOT  AllPortsSameDT=off
  Unit Delay : UnitDelay  SampleTime=-1
  Q : Outport
  !Q : Outport  Port=2
  wires:
  S/1 -> Logical Operator2/1
  Rp/1 -> Logical Operator/1
  Logical Operator3/1 -> !Q/1
  Unit Delay/1 -> Logical Operator2/2
  Logical Operator1/1 -> Unit Delay/1, Logical Operator3/1, Q/1
  Logical Operator2/1 -> Logical Operator1/2
  Logical Operator/1 -> Logical Operator1/1

== system EmE_MBD_Blockset/User-Defined Functions/Snoop/CCP_ETC_SS1/Signal Data Pairing/Update Signal12/Reset Logic ==
  CurrentPID : Inport
  ResetDAQ : Inport  Port=2
  CCP_SNOOP_DAQSIZE : Constant  Value=16  OutDataTypeStr=uint8
  CCP_SNOOP_FIRSTPID : Constant  Value=64  OutDataTypeStr=uint8
  Divide : Product  Inputs=*/
  Logical Operator : Logic  Operator=OR  AllPortsSameDT=off  OutDataTypeStr=boolean
  Relational Operator : RelationalOperator  Operator===  OutDataTypeStr=boolean  RndMeth=Nearest
  Relational Operator1 : RelationalOperator  Operator===  OutDataTypeStr=boolean  RndMeth=Nearest
  Reset ALL : Constant  Value=250  OutDataTypeStr=uint8
  Subtract : Sum  Inputs=+-
  Reset : Outport
  wires:
  CCP_SNOOP_FIRSTPID/1 -> Subtract/2
  Logical Operator/1 -> Reset/1
  Relational Operator1/1 -> Logical Operator/2
  Relational Operator/1 -> Logical Operator/1
  Reset ALL/1 -> Relational Operator1/2
  ResetDAQ/1 -> Relational Operator1/1, Relational Operator/2
  Divide/1 -> Relational Operator/1  "CurrentDAQ"
  CCP_SNOOP_DAQSIZE/1 -> Divide/2
  Subtract/1 -> Divide/1
  CurrentPID/1 -> Subtract/1

== system EmE_MBD_Blockset/User-Defined Functions/Snoop/CCP_ETC_SS1/Signal Data Pairing/Update Signal2/Latch w Update ==
  f_update : Inport
  In : Inport  Port=2
  Switch : Switch  Criteria=u2 ~= 0
  Unit Delay1 : UnitDelay  SampleTime=-1
  Latched : Outport
  wires:
  Unit Delay1/1 -> Switch/3
  Switch/1 -> Unit Delay1/1, Latched/1
  In/1 -> Switch/1
  f_update/1 -> Switch/2

== system EmE_MBD_Blockset/User-Defined Functions/Snoop/CCP_ETC_SS1/Signal Data Pairing/Update Signal2/Latch w Update1 ==
  f_update : Inport
  In : Inport  Port=2
  Switch : Switch  Criteria=u2 ~= 0
  Unit Delay1 : UnitDelay  SampleTime=-1
  Latched : Outport
  wires:
  f_update/1 -> Switch/2
  In/1 -> Switch/1
  Switch/1 -> Latched/1, Unit Delay1/1
  Unit Delay1/1 -> Switch/3

== system EmE_MBD_Blockset/User-Defined Functions/Snoop/CCP_ETC_SS1/Signal Data Pairing/Update Signal2/RS Flop-Flop Rp ==
  Rp : Inport
  S : Inport  Port=2
  Logical Operator : Logic  Operator=NOT  AllPortsSameDT=off
  Logical Operator1 : Logic  AllPortsSameDT=off
  Logical Operator2 : Logic  Operator=OR  AllPortsSameDT=off
  Logical Operator3 : Logic  Operator=NOT  AllPortsSameDT=off
  Unit Delay : UnitDelay  SampleTime=-1
  Q : Outport
  !Q : Outport  Port=2
  wires:
  S/1 -> Logical Operator2/1
  Rp/1 -> Logical Operator/1
  Logical Operator3/1 -> !Q/1
  Unit Delay/1 -> Logical Operator2/2
  Logical Operator1/1 -> Unit Delay/1, Logical Operator3/1, Q/1
  Logical Operator2/1 -> Logical Operator1/2
  Logical Operator/1 -> Logical Operator1/1

== system EmE_MBD_Blockset/User-Defined Functions/Snoop/CCP_ETC_SS1/Signal Data Pairing/Update Signal2/Reset Logic ==
  CurrentPID : Inport
  ResetDAQ : Inport  Port=2
  CCP_SNOOP_DAQSIZE : Constant  Value=16  OutDataTypeStr=uint8
  CCP_SNOOP_FIRSTPID : Constant  Value=64  OutDataTypeStr=uint8
  Divide : Product  Inputs=*/
  Logical Operator : Logic  Operator=OR  AllPortsSameDT=off  OutDataTypeStr=boolean
  Relational Operator : RelationalOperator  Operator===  OutDataTypeStr=boolean  RndMeth=Nearest
  Relational Operator1 : RelationalOperator  Operator===  OutDataTypeStr=boolean  RndMeth=Nearest
  Reset ALL : Constant  Value=250  OutDataTypeStr=uint8
  Subtract : Sum  Inputs=+-
  Reset : Outport
  wires:
  CCP_SNOOP_FIRSTPID/1 -> Subtract/2
  Logical Operator/1 -> Reset/1
  Relational Operator1/1 -> Logical Operator/2
  Relational Operator/1 -> Logical Operator/1
  Reset ALL/1 -> Relational Operator1/2
  ResetDAQ/1 -> Relational Operator1/1, Relational Operator/2
  Divide/1 -> Relational Operator/1  "CurrentDAQ"
  CCP_SNOOP_DAQSIZE/1 -> Divide/2
  Subtract/1 -> Divide/1
  CurrentPID/1 -> Subtract/1

== system EmE_MBD_Blockset/User-Defined Functions/Snoop/CCP_ETC_SS1/Signal Data Pairing/Update Signal3/Latch w Update ==
  f_update : Inport
  In : Inport  Port=2
  Switch : Switch  Criteria=u2 ~= 0
  Unit Delay1 : UnitDelay  SampleTime=-1
  Latched : Outport
  wires:
  Unit Delay1/1 -> Switch/3
  Switch/1 -> Unit Delay1/1, Latched/1
  In/1 -> Switch/1
  f_update/1 -> Switch/2

== system EmE_MBD_Blockset/User-Defined Functions/Snoop/CCP_ETC_SS1/Signal Data Pairing/Update Signal3/Latch w Update1 ==
  f_update : Inport
  In : Inport  Port=2
  Switch : Switch  Criteria=u2 ~= 0
  Unit Delay1 : UnitDelay  SampleTime=-1
  Latched : Outport
  wires:
  f_update/1 -> Switch/2
  In/1 -> Switch/1
  Switch/1 -> Latched/1, Unit Delay1/1
  Unit Delay1/1 -> Switch/3

== system EmE_MBD_Blockset/User-Defined Functions/Snoop/CCP_ETC_SS1/Signal Data Pairing/Update Signal3/RS Flop-Flop Rp ==
  Rp : Inport
  S : Inport  Port=2
  Logical Operator : Logic  Operator=NOT  AllPortsSameDT=off
  Logical Operator1 : Logic  AllPortsSameDT=off
  Logical Operator2 : Logic  Operator=OR  AllPortsSameDT=off
  Logical Operator3 : Logic  Operator=NOT  AllPortsSameDT=off
  Unit Delay : UnitDelay  SampleTime=-1
  Q : Outport
  !Q : Outport  Port=2
  wires:
  S/1 -> Logical Operator2/1
  Rp/1 -> Logical Operator/1
  Logical Operator3/1 -> !Q/1
  Unit Delay/1 -> Logical Operator2/2
  Logical Operator1/1 -> Unit Delay/1, Logical Operator3/1, Q/1
  Logical Operator2/1 -> Logical Operator1/2
  Logical Operator/1 -> Logical Operator1/1

== system EmE_MBD_Blockset/User-Defined Functions/Snoop/CCP_ETC_SS1/Signal Data Pairing/Update Signal3/Reset Logic ==
  CurrentPID : Inport
  ResetDAQ : Inport  Port=2
  CCP_SNOOP_DAQSIZE : Constant  Value=16  OutDataTypeStr=uint8
  CCP_SNOOP_FIRSTPID : Constant  Value=64  OutDataTypeStr=uint8
  Divide : Product  Inputs=*/
  Logical Operator : Logic  Operator=OR  AllPortsSameDT=off  OutDataTypeStr=boolean
  Relational Operator : RelationalOperator  Operator===  OutDataTypeStr=boolean  RndMeth=Nearest
  Relational Operator1 : RelationalOperator  Operator===  OutDataTypeStr=boolean  RndMeth=Nearest
  Reset ALL : Constant  Value=250  OutDataTypeStr=uint8
  Subtract : Sum  Inputs=+-
  Reset : Outport
  wires:
  CCP_SNOOP_FIRSTPID/1 -> Subtract/2
  Logical Operator/1 -> Reset/1
  Relational Operator1/1 -> Logical Operator/2
  Relational Operator/1 -> Logical Operator/1
  Reset ALL/1 -> Relational Operator1/2
  ResetDAQ/1 -> Relational Operator1/1, Relational Operator/2
  Divide/1 -> Relational Operator/1  "CurrentDAQ"
  CCP_SNOOP_DAQSIZE/1 -> Divide/2
  Subtract/1 -> Divide/1
  CurrentPID/1 -> Subtract/1

== system EmE_MBD_Blockset/User-Defined Functions/Snoop/CCP_ETC_SS1/Signal Data Pairing/Update Signal4/Latch w Update ==
  f_update : Inport
  In : Inport  Port=2
  Switch : Switch  Criteria=u2 ~= 0
  Unit Delay1 : UnitDelay  SampleTime=-1
  Latched : Outport
  wires:
  Unit Delay1/1 -> Switch/3
  Switch/1 -> Unit Delay1/1, Latched/1
  In/1 -> Switch/1
  f_update/1 -> Switch/2

== system EmE_MBD_Blockset/User-Defined Functions/Snoop/CCP_ETC_SS1/Signal Data Pairing/Update Signal4/Latch w Update1 ==
  f_update : Inport
  In : Inport  Port=2
  Switch : Switch  Criteria=u2 ~= 0
  Unit Delay1 : UnitDelay  SampleTime=-1
  Latched : Outport
  wires:
  f_update/1 -> Switch/2
  In/1 -> Switch/1
  Switch/1 -> Latched/1, Unit Delay1/1
  Unit Delay1/1 -> Switch/3

== system EmE_MBD_Blockset/User-Defined Functions/Snoop/CCP_ETC_SS1/Signal Data Pairing/Update Signal4/RS Flop-Flop Rp ==
  Rp : Inport
  S : Inport  Port=2
  Logical Operator : Logic  Operator=NOT  AllPortsSameDT=off
  Logical Operator1 : Logic  AllPortsSameDT=off
  Logical Operator2 : Logic  Operator=OR  AllPortsSameDT=off
  Logical Operator3 : Logic  Operator=NOT  AllPortsSameDT=off
  Unit Delay : UnitDelay  SampleTime=-1
  Q : Outport
  !Q : Outport  Port=2
  wires:
  S/1 -> Logical Operator2/1
  Rp/1 -> Logical Operator/1
  Logical Operator3/1 -> !Q/1
  Unit Delay/1 -> Logical Operator2/2
  Logical Operator1/1 -> Unit Delay/1, Logical Operator3/1, Q/1
  Logical Operator2/1 -> Logical Operator1/2
  Logical Operator/1 -> Logical Operator1/1

== system EmE_MBD_Blockset/User-Defined Functions/Snoop/CCP_ETC_SS1/Signal Data Pairing/Update Signal4/Reset Logic ==
  CurrentPID : Inport
  ResetDAQ : Inport  Port=2
  CCP_SNOOP_DAQSIZE : Constant  Value=16  OutDataTypeStr=uint8
  CCP_SNOOP_FIRSTPID : Constant  Value=64  OutDataTypeStr=uint8
  Divide : Product  Inputs=*/
  Logical Operator : Logic  Operator=OR  AllPortsSameDT=off  OutDataTypeStr=boolean
  Relational Operator : RelationalOperator  Operator===  OutDataTypeStr=boolean  RndMeth=Nearest
  Relational Operator1 : RelationalOperator  Operator===  OutDataTypeStr=boolean  RndMeth=Nearest
  Reset ALL : Constant  Value=250  OutDataTypeStr=uint8
  Subtract : Sum  Inputs=+-
  Reset : Outport
  wires:
  CCP_SNOOP_FIRSTPID/1 -> Subtract/2
  Logical Operator/1 -> Reset/1
  Relational Operator1/1 -> Logical Operator/2
  Relational Operator/1 -> Logical Operator/1
  Reset ALL/1 -> Relational Operator1/2
  ResetDAQ/1 -> Relational Operator1/1, Relational Operator/2
  Divide/1 -> Relational Operator/1  "CurrentDAQ"
  CCP_SNOOP_DAQSIZE/1 -> Divide/2
  Subtract/1 -> Divide/1
  CurrentPID/1 -> Subtract/1

== system EmE_MBD_Blockset/User-Defined Functions/Snoop/CCP_ETC_SS1/Signal Data Pairing/Update Signal5/Latch w Update ==
  f_update : Inport
  In : Inport  Port=2
  Switch : Switch  Criteria=u2 ~= 0
  Unit Delay1 : UnitDelay  SampleTime=-1
  Latched : Outport
  wires:
  Unit Delay1/1 -> Switch/3
  Switch/1 -> Unit Delay1/1, Latched/1
  In/1 -> Switch/1
  f_update/1 -> Switch/2

== system EmE_MBD_Blockset/User-Defined Functions/Snoop/CCP_ETC_SS1/Signal Data Pairing/Update Signal5/Latch w Update1 ==
  f_update : Inport
  In : Inport  Port=2
  Switch : Switch  Criteria=u2 ~= 0
  Unit Delay1 : UnitDelay  SampleTime=-1
  Latched : Outport
  wires:
  f_update/1 -> Switch/2
  In/1 -> Switch/1
  Switch/1 -> Latched/1, Unit Delay1/1
  Unit Delay1/1 -> Switch/3

== system EmE_MBD_Blockset/User-Defined Functions/Snoop/CCP_ETC_SS1/Signal Data Pairing/Update Signal5/RS Flop-Flop Rp ==
  Rp : Inport
  S : Inport  Port=2
  Logical Operator : Logic  Operator=NOT  AllPortsSameDT=off
  Logical Operator1 : Logic  AllPortsSameDT=off
  Logical Operator2 : Logic  Operator=OR  AllPortsSameDT=off
  Logical Operator3 : Logic  Operator=NOT  AllPortsSameDT=off
  Unit Delay : UnitDelay  SampleTime=-1
  Q : Outport
  !Q : Outport  Port=2
  wires:
  S/1 -> Logical Operator2/1
  Rp/1 -> Logical Operator/1
  Logical Operator3/1 -> !Q/1
  Unit Delay/1 -> Logical Operator2/2
  Logical Operator1/1 -> Unit Delay/1, Logical Operator3/1, Q/1
  Logical Operator2/1 -> Logical Operator1/2
  Logical Operator/1 -> Logical Operator1/1

== system EmE_MBD_Blockset/User-Defined Functions/Snoop/CCP_ETC_SS1/Signal Data Pairing/Update Signal5/Reset Logic ==
  CurrentPID : Inport
  ResetDAQ : Inport  Port=2
  CCP_SNOOP_DAQSIZE : Constant  Value=16  OutDataTypeStr=uint8
  CCP_SNOOP_FIRSTPID : Constant  Value=64  OutDataTypeStr=uint8
  Divide : Product  Inputs=*/
  Logical Operator : Logic  Operator=OR  AllPortsSameDT=off  OutDataTypeStr=boolean
  Relational Operator : RelationalOperator  Operator===  OutDataTypeStr=boolean  RndMeth=Nearest
  Relational Operator1 : RelationalOperator  Operator===  OutDataTypeStr=boolean  RndMeth=Nearest
  Reset ALL : Constant  Value=250  OutDataTypeStr=uint8
  Subtract : Sum  Inputs=+-
  Reset : Outport
  wires:
  CCP_SNOOP_FIRSTPID/1 -> Subtract/2
  Logical Operator/1 -> Reset/1
  Relational Operator1/1 -> Logical Operator/2
  Relational Operator/1 -> Logical Operator/1
  Reset ALL/1 -> Relational Operator1/2
  ResetDAQ/1 -> Relational Operator1/1, Relational Operator/2
  Divide/1 -> Relational Operator/1  "CurrentDAQ"
  CCP_SNOOP_DAQSIZE/1 -> Divide/2
  Subtract/1 -> Divide/1
  CurrentPID/1 -> Subtract/1

== system EmE_MBD_Blockset/User-Defined Functions/Snoop/CCP_ETC_SS1/Signal Data Pairing/Update Signal6/Latch w Update ==
  f_update : Inport
  In : Inport  Port=2
  Switch : Switch  Criteria=u2 ~= 0
  Unit Delay1 : UnitDelay  SampleTime=-1
  Latched : Outport
  wires:
  Unit Delay1/1 -> Switch/3
  Switch/1 -> Unit Delay1/1, Latched/1
  In/1 -> Switch/1
  f_update/1 -> Switch/2

== system EmE_MBD_Blockset/User-Defined Functions/Snoop/CCP_ETC_SS1/Signal Data Pairing/Update Signal6/Latch w Update1 ==
  f_update : Inport
  In : Inport  Port=2
  Switch : Switch  Criteria=u2 ~= 0
  Unit Delay1 : UnitDelay  SampleTime=-1
  Latched : Outport
  wires:
  f_update/1 -> Switch/2
  In/1 -> Switch/1
  Switch/1 -> Latched/1, Unit Delay1/1
  Unit Delay1/1 -> Switch/3

== system EmE_MBD_Blockset/User-Defined Functions/Snoop/CCP_ETC_SS1/Signal Data Pairing/Update Signal6/RS Flop-Flop Rp ==
  Rp : Inport
  S : Inport  Port=2
  Logical Operator : Logic  Operator=NOT  AllPortsSameDT=off
  Logical Operator1 : Logic  AllPortsSameDT=off
  Logical Operator2 : Logic  Operator=OR  AllPortsSameDT=off
  Logical Operator3 : Logic  Operator=NOT  AllPortsSameDT=off
  Unit Delay : UnitDelay  SampleTime=-1
  Q : Outport
  !Q : Outport  Port=2
  wires:
  S/1 -> Logical Operator2/1
  Rp/1 -> Logical Operator/1
  Logical Operator3/1 -> !Q/1
  Unit Delay/1 -> Logical Operator2/2
  Logical Operator1/1 -> Unit Delay/1, Logical Operator3/1, Q/1
  Logical Operator2/1 -> Logical Operator1/2
  Logical Operator/1 -> Logical Operator1/1
